simulink model "servo_model"  (R2016b)
settings: Solver=FixedStepDiscrete  StartTime=0.0  StopTime=inf  FixedStep=0.002  RelTol=1e-3  EnableMultiTasking=on
settings Model: ExtModeTrigDuration=10000  Creator=drbutt  LastModifiedBy=drbutt
settings SolverCC: PositivePriorityOrder=on
settings RTWCC: SystemTargetFile=quarc_win64.tlc  TemplateMakefile=quarc_default_tmf  Description=QUARC Win64 Target
settings STFCustomTargetCC: TargetPreCompLibLocation=C:\PROGRA~3\QUARC\lib\2016b\win64\release  TargetLangStandard=C99 (ISO)  ConcurrentExecutionCompliant=on  SystemTargetFile=quarc_win64.tlc
settings GRTTargetCC: TargetPreCompLibLocation=C:\PROGRA~3\QUARC\lib\2016b\win64\release  ParMdlRefBuildCompliant=off  CompOptLevelCompliant=off  CombineOutputUpdateFcns=off  MatFileLogging=off  CPPClassGenCompliant=off  GRTInterface=on  UseToolchainInfoCompliant=off  ExtMode=on  ExtModeMexFile=quarc_comm

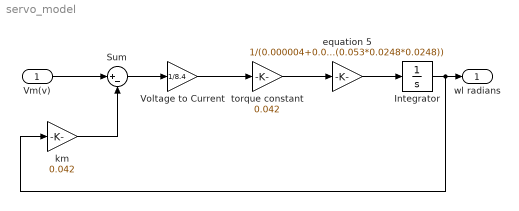
== system servo_model ==
  Vm(v) : Inport
  Integrator : Integrator
  Sum : Sum  Inputs=|+-
  "Voltage to Current " : Gain  Gain=1/8.4
  equation 5 : Gain  Gain=1/(0.000004+0.0000006+0.5*(0.053*0.0248*0.0248))
  "km " : Gain  Gain=0.042
  torque constant : Gain  Gain=0.042
  "wl radians " : Outport
  wires:
  Vm(v)/1 -> Sum/1
  "Voltage to Current "/1 -> torque constant/1
  Sum/1 -> "Voltage to Current "/1
  "km "/1 -> Sum/2
  torque constant/1 -> equation 5/1
  equation 5/1 -> Integrator/1
  Integrator/1 -> "km "/1, "wl radians "/1
